simulink model "Configurable_Carrier"  (Simulink 6.5)
settings: Solver=ode45  StartTime=0.0  StopTime=10.0  RelTol=1e-3
libraries: dspmathops x1, dspsigops x1
settings Model: Creator=Shay  LastModifiedBy=dsp

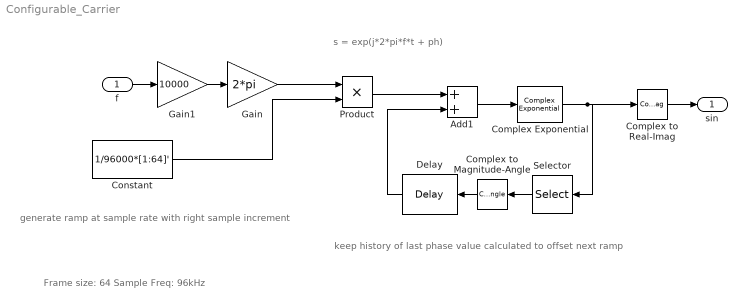
== system Configurable_Carrier ==
  note: keep history of last phase value calculated
      | to offset next ramp
  note: s = exp(j*2*pi*f*t + ph)
  note: generate ramp at sample rate
      | with right sample increment
  note: Frame size: 64
      | Sample Freq: 96kHz
  f : Inport
  Add1 : Sum  OutScaling=2^-10
  Complex Exponential : dspmathops/Complex Exponential  SystemSampleTime=-1
  Complex to Magnitude-Angle : ComplexToMagnitudeAngle  Orientation=left  Output=Angle
  Complex to Real-Imag : ComplexToRealImag  Output=Real
  Constant : Constant  Value=1/96000*[1:64]'  VectorParams1D=off  OutDataTypeMode=single  OutDataType=sfix(16)  ConRadixGroup=Use specified scaling  OutScaling=2^0  SampleTime=0.001  FramePeriod=64/96000
      settings: SamplingMode=Frame based
  Delay : dspsigops/Delay  Orientation=left  dly_unit=Samples  delay=1  ic_detail=off  dif_ic_for_ch=off  dif_ic_for_dly=off  ic=0  reset_popup=None
  Gain : Gain  Gain=2*pi
  Gain1 : Gain  Gain=10000
  Product : Product  RndMeth=Zero
  Selector : Selector  Orientation=left  InputType=Vector  ElementSrc=Internal  Elements=[64]  RowSrc=Internal  Rows=1  ColumnSrc=Internal  Columns=1  InputPortWidth=64  IndexIsStartValue=off
  sin : Outport
  wires:
  Gain1/1 -> Gain/1
  Complex to Real-Imag/1 -> sin/1
  Add1/1 -> Complex Exponential/1
  Product/1 -> Add1/1
  Delay/1 -> Add1/2
  Complex to Magnitude-Angle/1 -> Delay/1
  Selector/1 -> Complex to Magnitude-Angle/1
  Complex Exponential/1 -> Selector/1, Complex to Real-Imag/1
  Gain/1 -> Product/1
  Constant/1 -> Product/2
  f/1 -> Gain1/1
